simulink model "RF_TX_Model"  (R2026a)
settings: Solver=VariableStepAuto
InitFcn:
  | warning('off')
model workspace (MAT data in the model file):
  Az = 30
  phaseShifts = [20.1529923745; -88.4621483039; 162.922711018; 54.3075703392; -54.3075703392; -162.922711018; 88.4621483039; -20.1529923745]
values from neighbouring files (symbols this model uses):
  BW = 1e8    (= 100000000)    [MatchingNetworkDesign.m]    (also in analyzeReferenceRFBudget.m; build12GHzTransmitterRFBudget.m; build12GHzTransmitterRFBudget_Pin20dBm.m; buildReferenceRFBudgetAnalyzer.m)
  fIF = 4e9    (= 4000000000)    [analyze12GHzTransmitterBudget.m]    (also in analyzeReferenceRFBudget.m; build12GHzTransmitterRFBudget.m; build12GHzTransmitterRFBudget_Pin20dBm.m; buildReferenceRFBudgetAnalyzer.m)
  S = sparameters(rfAntenna,fRF)    [runAntenna2Bits.m]
  splitterCorporate = design(powerDividerCorporate(NumOutputPorts=N,SplitterElement=e), fRF)    [runAntenna2Bits.m]
undefined symbols (not defined in the file or in its folder): rational, sparameters
libraries: simrfV2elements x7, simrfV2_lib x6, dspstat3 x5, simrfV2util1 x3, commrflib2 x1, simrfV2systems x1, simrfV2private x1, dspmathops x1
(part 3 of 3)

== system RF_TX_Model/TX BFIC/Wilkinson Splitter/AuxData ==
